simulink model "DDEF_NYLON"  (R2026a)
settings: Solver=ode45  StopTime=10  MaxStep=1e-4  RelTol=1e-6
libraries: simulink x1
settings Model: Creator=Satyanarayan  LastModifiedBy=Satyanarayan

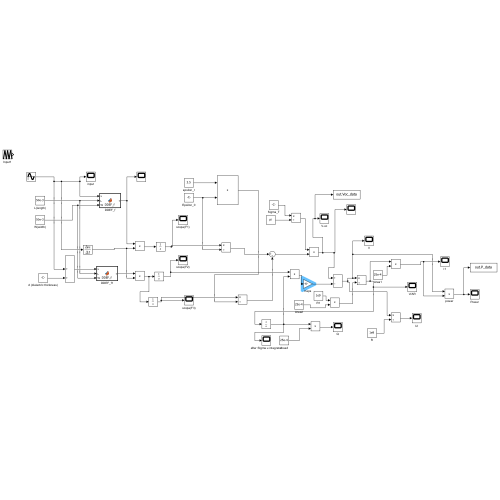
[thumbnail: Simulink's stored preview of the top-level diagram]
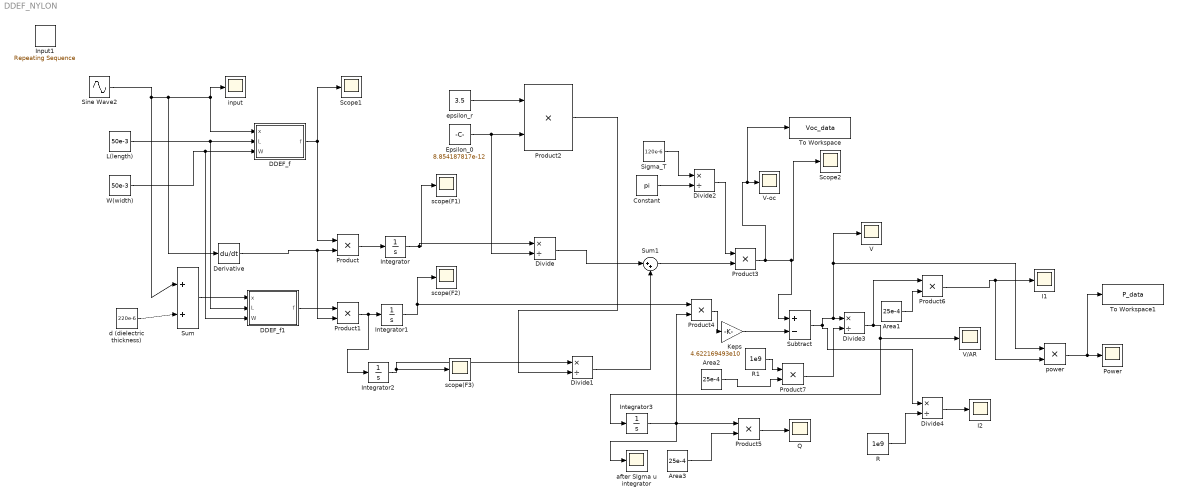
== system DDEF_NYLON ==
  Area1 : Constant  Value=25e-4
  Area2 : Constant  Value=25e-4
  Area3 : Constant  Value=25e-4
  Constant : Constant  Value=pi
  DDEF_f : MATLAB Function  TreatAsAtomicUnit=on
  DDEF_f1 : MATLAB Function  TreatAsAtomicUnit=on
  Derivative : Derivative
  Divide{,1..4} (5 alike) : Product  Inputs=*/
  Epsilon_0 : Constant  Value=8.854187817e-12
  I1 : Scope
      settings: ActiveDisplayYMinimum=-1  ActiveDisplayYMaximum=1  DataLoggingVariableName=ScopeData11
  I2 : Scope
      settings: ActiveDisplayYMinimum=-1  ActiveDisplayYMaximum=1  DataLoggingVariableName=ScopeData12
  Input1 : simulink/Sources/Repeating Sequence  rep_seq_t=[0 0.5 1]  rep_seq_y=[0 0.01 0]
  Integrator : Integrator
  Integrator1 : Integrator  InitialCondition=3.44206e-4
  Integrator2 : Integrator
  Integrator3 : Integrator
  Keps : Gain  Gain=4.622169493e10
  L(length) : Constant  Value=50e-3
  Power : Scope
      settings: ActiveDisplayYMinimum=-0.00046209975030593484  ActiveDisplayYMaximum=0.0041588977527534142  DataLoggingVariableName=ScopeData13
  Product{,1..7} (8 alike) : Product
  Q : Scope
      settings: ActiveDisplayYMinimum=-1  ActiveDisplayYMaximum=1  DataLoggingVariableName=ScopeData10
  R : Constant  Value=1e9
  R1 : Constant  Value=1e9
  Scope1 : Scope
      settings: ActiveDisplayYMinimum=0.392699081716402  ActiveDisplayYMaximum=1.7016960205353724
  Scope2 : Scope
      settings: ActiveDisplayYMinimum=-1  ActiveDisplayYMaximum=1  DataLoggingVariableName=ScopeData5
  Sigma_T : Constant  Value=120e-6
  Sine Wave2 : Sin  Amplitude=2.5e-3  Bias=2.5e-3  Frequency=2*pi  Phase=3*pi/2  SampleTime=0
  Subtract : Sum  Inputs=+-
  Sum : Sum  Inputs=|++
  Sum1 : Sum  Inputs=|++
  To Workspace : ToWorkspace  VariableName=Voc_data  SaveFormat=Timeseries  SampleTime=-1
  To Workspace1 : ToWorkspace  VariableName=P_data  SaveFormat=Timeseries  SampleTime=-1
  V : Scope
      settings: ActiveDisplayYMinimum=-1275.0051318724477  ActiveDisplayYMaximum=2278.0071328579675  DataLoggingVariableName=ScopeData6
  V-oc : Scope
      settings: ActiveDisplayYMinimum=-4819.8788285773553  ActiveDisplayYMaximum=43269.459838287345  DataLoggingVariableName=ScopeData9
  V/AR : Scope
      settings: ActiveDisplayYMinimum=-1  ActiveDisplayYMaximum=1  DataLoggingVariableName=ScopeData8
  W(width) : Constant  Value=50e-3
  after SIgma u integrator : Scope
      settings: ActiveDisplayYMinimum=-3.4716855225550229E-6  ActiveDisplayYMaximum=3.1245169702995217E-5  DataLoggingVariableName=ScopeData7
  d (dielectric thickness) : Constant  Value=220e-6
  epsilon_r : Constant  Value=3.5
  input : Scope
      settings: ActiveDisplayYMinimum=-0.0012499995532938208  ActiveDisplayYMaximum=0.011249995979644389
  power : Product
  scope(F1) : Scope
      settings: ActiveDisplayYMinimum=-0.00121173424121706  ActiveDisplayYMaximum=0.01090560817095354  DataLoggingVariableName=ScopeData2
  scope(F2) : Scope
      settings: ActiveDisplayYMinimum=0.00041232627300281824  ActiveDisplayYMaximum=0.01127511879777789  DataLoggingVariableName=ScopeData3
  scope(F3) : Scope
      settings: ActiveDisplayYMinimum=-0.0010878737269972396  ActiveDisplayYMaximum=0.009774918797777957  DataLoggingVariableName=ScopeData4
  wires:
  Area1/1 -> Product6/2
  Divide2/1 -> Product3/1
  Product4/1 -> Keps/1
  Divide4/1 -> I2/1
  Divide/1 -> Sum1/1
  Sigma_T/1 -> Divide2/1
  Keps/1 -> Subtract/2
  Divide3/1 -> Product6/1, Integrator3/1, V/AR/1
  Sum/1 -> DDEF_f1/1(x)
  d (dielectric thickness)/1 -> Sum/2
  Product/1 -> Integrator/1
  Derivative/1 -> Product1/2, Product/2
  Integrator/1 -> Divide/1, scope(F1)/1
  Product3/1 -> To Workspace/1, V-oc/1, Subtract/1, Scope2/1
  Constant/1 -> Divide2/2
  Product7/1 -> Divide3/2
  Integrator2/1 -> Divide1/1, scope(F3)/1
  Product5/1 -> Q/1
  Sine Wave2/1 -> Sum/1, Derivative/1, DDEF_f/1(x), input/1
  R/1 -> Divide4/2
  power/1 -> To Workspace1/1, Power/1
  Area3/1 -> Product5/2
  Integrator3/1 -> Product5/1, after SIgma u integrator/1, Product4/2
  Subtract/1 -> Divide4/1, V/1, power/1, Divide3/1
  Product1/1 -> Integrator2/1, Integrator1/1
  Product6/1 -> power/2, I1/1
  Product2/1 -> Divide1/2
  Divide1/1 -> Sum1/2
  L(length)/1 -> DDEF_f1/2(L), DDEF_f/2(L)
  Epsilon_0/1 -> Divide/2, Product2/2
  DDEF_f/1(f) -> Product/1, Scope1/1
  DDEF_f1/1(f) -> Product1/1
  Integrator1/1 -> Product4/1, scope(F2)/1
  Sum1/1 -> Product3/2
  W(width)/1 -> DDEF_f1/3(W), DDEF_f/3(W)
  epsilon_r/1 -> Product2/1
  R1/1 -> Product7/1
  Area2/1 -> Product7/2

== matlab function DDEF_NYLON/DDEF_f ==
  data: x input; f output; L input; W input
function f = DDEF_f(x,L,W)

z = max(x,1e-12);

f = atan((L*W)/(2*z*sqrt(L^2 + W^2 + 4*z^2)));

end

== matlab function DDEF_NYLON/DDEF_f1 ==
  data: x input; f output; L input; W input
function f = DDEF_f(x,L,W)

z = max(x,1e-12);

f = atan((L*W)/(2*z*sqrt(L^2 + W^2 + 4*z^2)));

end
